simulink library "vec_norm"  (R2020b)
settings: Solver=VariableStepAuto  StartTime=0.0  StopTime=10.0  RelTol=1e-3
settings Model: Creator=whitehole  LastModifiedBy=whitehole

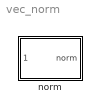
== system vec_norm ==
  norm : Subsystem

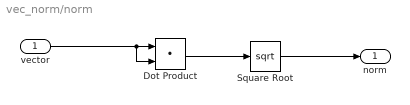
== system vec_norm/norm ==
  vector : Inport
  Dot Product : DotProduct  InputSameDT=on  OutDataTypeStr=Inherit: Inherit via internal rule
  Square Root : Sqrt  SaturateOnIntegerOverflow=on
  norm : Outport
  wires:
  Dot Product/1 -> Square Root/1
  vector/1 -> Dot Product/2, Dot Product/1
  Square Root/1 -> norm/1
